simulink model "butterfly"  (R2020a)
settings: Solver=VariableStepAuto  StartTime=0.0  StopTime=10.0  RelTol=1e-3
settings Model: Creator=g-oft  LastModifiedBy=g-oft

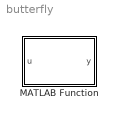
== system butterfly ==
  MATLAB Function : MATLAB Function  TreatAsAtomicUnit=on

== matlab function butterfly/MATLAB Function ==
  data: u input; y output
function y = fcn(u)
    bf = butterfly_robot(true);
y = u;
